simulink model "Sim_LabVaja1_4_1"  (R2019b)
settings: Solver=VariableStepAuto  StartTime=0.0  StopTime=1600  FixedStep=10  RelTol=1e-3
values from neighbouring files (symbols this model uses):
  CH1 = ro * S1    (= 10)    [LaboratorijskaVaja1_1.m]    (also in LaboratorijskaVaja1_2_3.m; LaboratorijskaVaja1_4.m; odvod.m)
  CH2 = ro * S2    (= 10)    [LaboratorijskaVaja1_1.m]    (also in LaboratorijskaVaja1_2_3.m; LaboratorijskaVaja1_4.m; odvod.m)
  RH1 = 5    [LaboratorijskaVaja1_1.m]    (also in LaboratorijskaVaja1_2_3.m; LaboratorijskaVaja1_4.m)
  RH2 = 10    [LaboratorijskaVaja1_1.m]    (also in LaboratorijskaVaja1_2_3.m; LaboratorijskaVaja1_4.m)
settings Model: Creator=bonce  LastModifiedBy=bonce
settings DataIOCC: ReturnWorkspaceOutputs=off

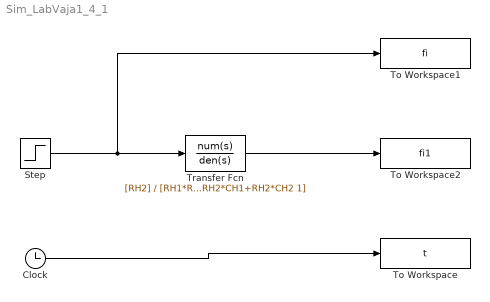
== system Sim_LabVaja1_4_1 ==
  Clock : Clock
  Step : Step  Time=0  After=0.02  SampleTime=15
  To Workspace : ToWorkspace  VariableName=t  SampleTime=-1
  To Workspace1 : ToWorkspace  VariableName=fi  SampleTime=-1
  To Workspace2 : ToWorkspace  VariableName=fi1  SampleTime=-1
  Transfer Fcn : TransferFcn  Numerator=[RH2]  Denominator=[RH1*RH2*CH1*CH2 RH1*CH1+RH2*CH1+RH2*CH2 1]  ContinuousStateAttributes='G2'
  wires:
  Step/1 -> To Workspace1/1, Transfer Fcn/1
  Transfer Fcn/1 -> To Workspace2/1
  Clock/1 -> To Workspace/1
